simulink library "Word2Bytes_lib"  (Simulink 8.1)
settings: Solver=ode45  StartTime=0.0  StopTime=10.0  RelTol=1e-3
settings Model: Creator=ch24070  LastModifiedBy=ch24070

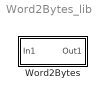
== system Word2Bytes_lib ==
  Word2Bytes : Subsystem

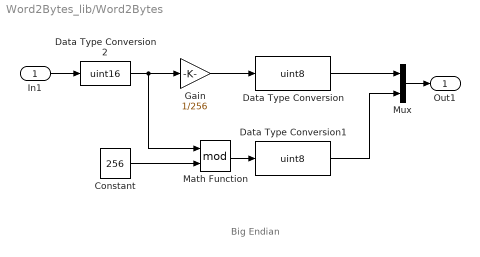
== system Word2Bytes_lib/Word2Bytes ==
  note: Big Endian
  In1 : Inport
  Constant : Constant  Value=256  OutDataTypeStr=uint16
  Data Type Conversion : DataTypeConversion  OutDataTypeStr=uint8
  Data Type Conversion1 : DataTypeConversion  OutDataTypeStr=uint8
  Data Type Conversion2 : DataTypeConversion  OutDataTypeStr=uint16
  Gain : Gain  Gain=1/256
  Math Function : Math  Operator=mod  SaturateOnIntegerOverflow=on
  Mux : Mux  Inputs=2
  Out1 : Outport
  wires:
  Data Type Conversion1/1 -> Mux/2
  Data Type Conversion/1 -> Mux/1
  Mux/1 -> Out1/1
  Math Function/1 -> Data Type Conversion1/1
  In1/1 -> Data Type Conversion2/1
  Constant/1 -> Math Function/2
  Gain/1 -> Data Type Conversion/1
  Data Type Conversion2/1 -> Gain/1, Math Function/1
